simulink model "Traj2"  (R2025b)
settings: Solver=VariableStepAuto  StartTime=0.0  StopTime=T_end  RelTol=1e-3
values from neighbouring files (symbols this model uses):
  K = lqr(A, B, Q, R)    [lq.m]    (also in lqr.m = lqr(A,B,Q,R))
  L = 0.4    [lq.m]    (also in lqr.m = 0.2)
  P = double(P)    [lq.m]    (also in lqr.m)
  theta0 = double(theta0)    [lq.m]    (also in lqr.m)
  theta_ref_unwrapped = double(theta_ref_unwrapped(:))    [lq.m]
  Ts_ref = double(Ts_ref)    [lq.m]    (also in lqr.m)
  vd_ref = double(vd_ref(:))    [lq.m]    (also in lqr.m)
  wd_ref = double(wd_ref(:))    [lq.m]    (also in lqr.m)
  x0 = double(x0)    [lq.m]    (also in lqr.m)
  y0 = double(y0)    [lq.m]    (also in lqr.m)
libraries: slpidlib x2
settings Model: Creator=mwali  LastModifiedBy=mwali

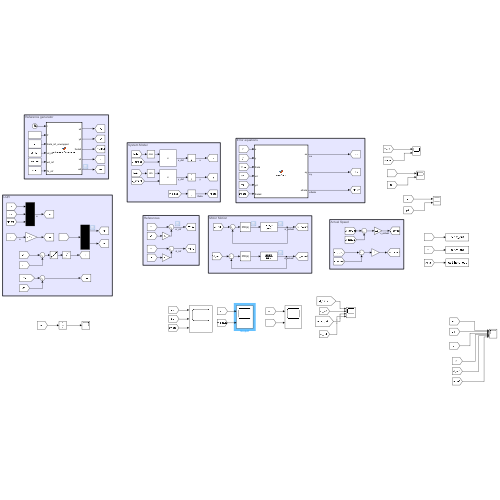
[thumbnail: Simulink's stored preview of the top-level diagram]
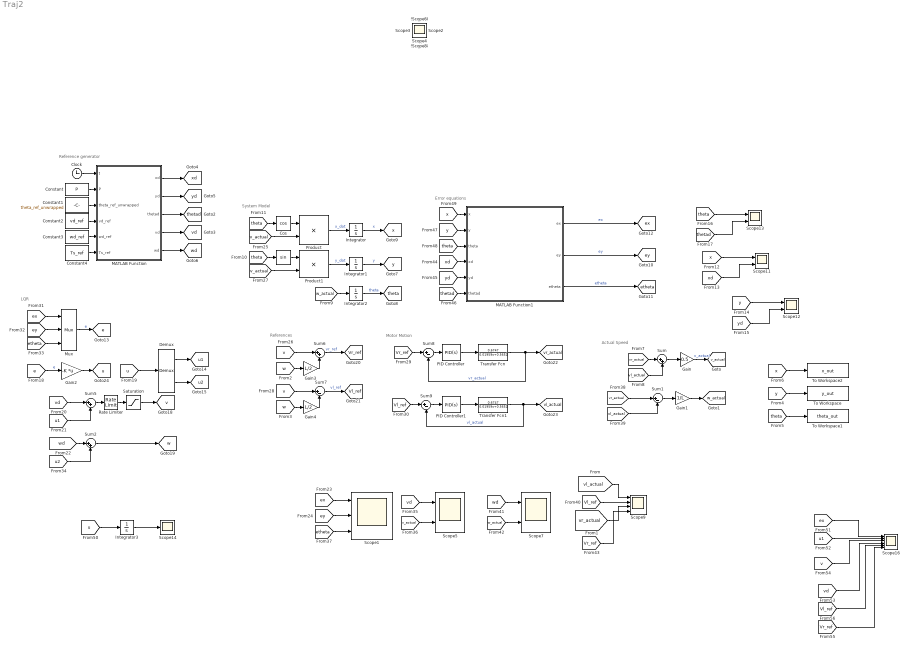
== system Traj2 ==
  note: Error equations
  note: Actual Speed
  note: Motor Motion
  note: References
  note: LQR
  note: System Model
  note: Reference generator
  " " : Trigonometry
  Clock : Clock
  Constant : Constant  Value=P
  Constant1 : Constant  Value=theta_ref_unwrapped
  Constant2 : Constant  Value=vd_ref
  Constant3 : Constant  Value=wd_ref
  Constant4 : Constant  Value=Ts_ref
  Cos : Trigonometry  Operator=cos
  Demux : Demux  Outputs=2
  Gain : Gain  Gain=0.5
  Gain1 : Gain  Gain=1/L
  Gain2 : Gain  Gain=-K  Multiplication=Matrix(K*u)
  Gain3 : Gain  Gain=L/2
  Gain4 : Gain  Gain=L/2
  Integrator : Integrator  InitialCondition=x0
  Integrator1 : Integrator  InitialCondition=y0
  Integrator2 : Integrator  InitialCondition=theta0
  Integrator3 : Integrator
  MATLAB Function : MATLAB Function  TreatAsAtomicUnit=on
  MATLAB Function1 : MATLAB Function  TreatAsAtomicUnit=on
  Mux : Mux  Inputs=3
  PID Controller : slpidlib/PID Controller  Controller=PID  Form=Parallel  TimeDomain=Continuous-time  UseExternalTs=off  SampleTime=-1  IntegratorMethod=Forward Euler  FilterMethod=Forward Euler  ControllerParametersSource=internal  P=4  I=0.05  UseKiTs=off  D=0  UseExternalDerivativeSource=off  N=100  UseFilter=on  TunerSelectOption=Transfer Function Based (PID Tuner App)  InitialConditionSource=internal  InitialConditionForIntegrator=0  InitialConditionForFilter=0  DifferentiatorICPrevScaledInput=0  ExternalReset=none  TrackingMode=off  Kt=1  LimitOutput=off  SatLimitsSource=internal  UpperSaturationLimit=0.5  LowerSaturationLimit=0  LinearizeAsGain=on  AntiWindupMode=clamping  Kb=1  LimitIntegrator=off  UpperIntegratorSaturationLimit=inf  LowerIntegratorSaturationLimit=-inf  POutMin=[]  POutMax=[]  IOutMin=[]  IOutMax=[]  DOutMin=[]  DOutMax=[]  NOutMin=[]  NOutMax=[]  SumOutMin=[]  SumOutMax=[]  SaturationOutMin=[]  SaturationOutMax=[]  PParamMin=[]  PParamMax=[]  IParamMin=[]  IParamMax=[]  DParamMin=[]  DParamMax=[]  NParamMin=[]  NParamMax=[]  KbParamMin=[]  KbParamMax=[]  KtParamMin=[]  KtParamMax=[]  KbOutMin=[]  KbOutMax=[]  KtOutMin=[]  KtOutMax=[]  IntegratorOutMin=[]  IntegratorOutMax=[]  FilterOutMin=[]  FilterOutMax=[]  SumI1OutMin=[]  SumI1OutMax=[]  SumI2OutMin=[]  SumI2OutMax=[]  SumI3OutMin=[]  SumI3OutMax=[]  SumI4OutMin=[]  SumI4OutMax=[]  SumDOutMin=[]  SumDOutMax=[]  DifferentiatorOutMin=[]  DifferentiatorOutMax=[]  FilterDiffOutCoefMin=[]  FilterDiffOutCoefMax=[]  ReciprocalOutMin=[]  ReciprocalOutMax=[]  SumDenOutMin=[]  SumDenOutMax=[]  SumNumOutMin=[]  SumNumOutMax=[]  DivideOutMin=[]  DivideOutMax=[]  UdiffTsProdOutMin=[]  UdiffTsProdOutMax=[]  NTsProdOutMin=[]  NTsProdOutMax=[]  UintegralTsProdOutMin=[]  UintegralTsProdOutMax=[]  UngainTsProdOutMin=[]  UngainTsProdOutMax=[]  ClampingZeroOutDataTypeStr=Inherit: Inherit via back propagation  ClampingZeroOutMin=[]  ClampingZeroOutMax=[]  FilterDenConstantOutDataTypeStr=Inherit: Inherit via back propagation  FilterDenConstantOutMin=[]  FilterDenConstantOutMax=[]  PCopyOutDataTypeStr=Inherit: Inherit via back propagation  PCopyOutMin=[]  PCopyOutMax=[]  NCopyOutDataTypeStr=Inherit: Inherit via back propagation  NCopyOutMin=[]  NCopyOutMax=[]  IntegratorContinuousStateAttributes=''  IntegratorStateMustResolveToSignalObject=off  IntegratorRTWStateStorageClass=Auto  FilterContinuousStateAttributes=''  FilterStateMustResolveToSignalObject=off  FilterRTWStateStorageClass=Auto  ParallelPVariant=InternalParameters  IdealPVariant=Disabled  IVariant=InternalParameters  DVariant=InternalParameters  IntegratorVariant=Continuous  SatVariant=Disabled  AWVariant=Passthrough  PCopyVariant=Disabled  TRVariant=Disabled  FdbkBlocksVariant=Forward  IdealPFdbkVariant=Disabled  SatFdbkVariant=Disabled  DerivativeFilterVariant=ContFilter  NVariant=InternalParameters  NCopyVariant=Disabled  FilterICVariant=InternalICsFilter  IntegratorICVariant=InternalICs  ExternalResetVariant=Disabled  TRSumVariant=Passthrough  SumFdbkVariant=Disabled  SumVariant=Sum_PID  TsampFilterVariant=InternalTs  TsampNgainVariant=Passthrough  TsampIntegralVariant=Disabled_SignalSpec  ExternalSaturationOutDataTypeStr=Inherit: Same as second input  DerivativeSourceVariant=ErrorSignal  PreIntVariant=InternalPreInt
  PID Controller1 : slpidlib/PID Controller  Controller=PID  Form=Parallel  TimeDomain=Continuous-time  UseExternalTs=off  SampleTime=-1  IntegratorMethod=Forward Euler  FilterMethod=Forward Euler  ControllerParametersSource=internal  P=4  I=0.05  UseKiTs=off  D=0  UseExternalDerivativeSource=off  N=100  UseFilter=on  TunerSelectOption=Transfer Function Based (PID Tuner App)  InitialConditionSource=internal  InitialConditionForIntegrator=0  InitialConditionForFilter=0  DifferentiatorICPrevScaledInput=0  ExternalReset=none  TrackingMode=off  Kt=1  LimitOutput=off  SatLimitsSource=internal  UpperSaturationLimit=0.5  LowerSaturationLimit=0  LinearizeAsGain=on  AntiWindupMode=clamping  Kb=1  LimitIntegrator=off  UpperIntegratorSaturationLimit=inf  LowerIntegratorSaturationLimit=-inf  POutMin=[]  POutMax=[]  IOutMin=[]  IOutMax=[]  DOutMin=[]  DOutMax=[]  NOutMin=[]  NOutMax=[]  SumOutMin=[]  SumOutMax=[]  SaturationOutMin=[]  SaturationOutMax=[]  PParamMin=[]  PParamMax=[]  IParamMin=[]  IParamMax=[]  DParamMin=[]  DParamMax=[]  NParamMin=[]  NParamMax=[]  KbParamMin=[]  KbParamMax=[]  KtParamMin=[]  KtParamMax=[]  KbOutMin=[]  KbOutMax=[]  KtOutMin=[]  KtOutMax=[]  IntegratorOutMin=[]  IntegratorOutMax=[]  FilterOutMin=[]  FilterOutMax=[]  SumI1OutMin=[]  SumI1OutMax=[]  SumI2OutMin=[]  SumI2OutMax=[]  SumI3OutMin=[]  SumI3OutMax=[]  SumI4OutMin=[]  SumI4OutMax=[]  SumDOutMin=[]  SumDOutMax=[]  DifferentiatorOutMin=[]  DifferentiatorOutMax=[]  FilterDiffOutCoefMin=[]  FilterDiffOutCoefMax=[]  ReciprocalOutMin=[]  ReciprocalOutMax=[]  SumDenOutMin=[]  SumDenOutMax=[]  SumNumOutMin=[]  SumNumOutMax=[]  DivideOutMin=[]  DivideOutMax=[]  UdiffTsProdOutMin=[]  UdiffTsProdOutMax=[]  NTsProdOutMin=[]  NTsProdOutMax=[]  UintegralTsProdOutMin=[]  UintegralTsProdOutMax=[]  UngainTsProdOutMin=[]  UngainTsProdOutMax=[]  ClampingZeroOutDataTypeStr=Inherit: Inherit via back propagation  ClampingZeroOutMin=[]  ClampingZeroOutMax=[]  FilterDenConstantOutDataTypeStr=Inherit: Inherit via back propagation  FilterDenConstantOutMin=[]  FilterDenConstantOutMax=[]  PCopyOutDataTypeStr=Inherit: Inherit via back propagation  PCopyOutMin=[]  PCopyOutMax=[]  NCopyOutDataTypeStr=Inherit: Inherit via back propagation  NCopyOutMin=[]  NCopyOutMax=[]  IntegratorContinuousStateAttributes=''  IntegratorStateMustResolveToSignalObject=off  IntegratorRTWStateStorageClass=Auto  FilterContinuousStateAttributes=''  FilterStateMustResolveToSignalObject=off  FilterRTWStateStorageClass=Auto  ParallelPVariant=InternalParameters  IdealPVariant=Disabled  IVariant=InternalParameters  DVariant=InternalParameters  IntegratorVariant=Continuous  SatVariant=Disabled  AWVariant=Passthrough  PCopyVariant=Disabled  TRVariant=Disabled  FdbkBlocksVariant=Forward  IdealPFdbkVariant=Disabled  SatFdbkVariant=Disabled  DerivativeFilterVariant=ContFilter  NVariant=InternalParameters  NCopyVariant=Disabled  FilterICVariant=InternalICsFilter  IntegratorICVariant=InternalICs  ExternalResetVariant=Disabled  TRSumVariant=Passthrough  SumFdbkVariant=Disabled  SumVariant=Sum_PID  TsampFilterVariant=InternalTs  TsampNgainVariant=Passthrough  TsampIntegralVariant=Disabled_SignalSpec  ExternalSaturationOutDataTypeStr=Inherit: Same as second input  DerivativeSourceVariant=ErrorSignal  PreIntVariant=InternalPreInt
  Product : Product
  Product1 : Product
  Rate Limiter : RateLimiter  RisingSlewLimit=0.1  FallingSlewLimit=-0.35  SampleTimeMode=inherited
  Saturation : Saturate  UpperLimit=0.3  LowerLimit=0
  Scope1 : Scope  NumInputPorts=3
      settings: ActiveDisplayYMinimum=-0.19694  ActiveDisplayYMaximum=0.26619
  Scope{5,7,11..13} (5 alike) : Scope  NumInputPorts=2
      Scope11 settings: ActiveDisplayYMinimum=-1  ActiveDisplayYMaximum=1  DataLoggingVariableName=ScopeData11
      Scope12 settings: ActiveDisplayYMinimum=-1  ActiveDisplayYMaximum=1  DataLoggingVariableName=ScopeData12
      Scope13 settings: ActiveDisplayYMinimum=1.0311287515557852  ActiveDisplayYMaximum=3.7167864278411562  DataLoggingVariableName=ScopeData13
      Scope5 settings: ActiveDisplayYMinimum=-0.041698068879938432  ActiveDisplayYMaximum=0.34024051073415013  DataLoggingVariableName=ScopeData5
      Scope7 settings: ActiveDisplayYMinimum=-2.7766  ActiveDisplayYMaximum=4.0045  DataLoggingVariableName=ScopeData7
  Scope{,2..4,6,8,10,14..15} (9 alike) : Scope
      Scope14 settings: ActiveDisplayYMinimum=-1  ActiveDisplayYMaximum=1  DataLoggingVariableName=ScopeData14
      Scope settings: ActiveDisplayYMinimum=-0.11929  ActiveDisplayYMaximum=0.80552
      Scope10 settings: ActiveDisplayYMinimum=-1  ActiveDisplayYMaximum=1  DataLoggingVariableName=ScopeData10
      Scope15 settings: ActiveDisplayYMinimum=-1  ActiveDisplayYMaximum=1  DataLoggingVariableName=ScopeData15
      Scope2 settings: ActiveDisplayYMinimum=-1  ActiveDisplayYMaximum=1  DataLoggingVariableName=ScopeData2
      Scope3 settings: ActiveDisplayYMinimum=-1  ActiveDisplayYMaximum=1  DataLoggingVariableName=ScopeData3
      Scope4 settings: ActiveDisplayYMinimum=-1  ActiveDisplayYMaximum=1  DataLoggingVariableName=ScopeData4
      Scope6 settings: ActiveDisplayYMinimum=-1  ActiveDisplayYMaximum=1  DataLoggingVariableName=ScopeData6
      Scope8 settings: ActiveDisplayYMinimum=-5.1687  ActiveDisplayYMaximum=3.6193  DataLoggingVariableName=ScopeData8
  Scope16 : Scope  NumInputPorts=6
      settings: ActiveDisplayYMinimum=-0.13161054609059852  ActiveDisplayYMaximum=0.33829750120743474  DataLoggingVariableName=ScopeData16
  Scope9 : Scope  NumInputPorts=4
      settings: ActiveDisplayYMinimum=-0.51559  ActiveDisplayYMaximum=1.245  DataLoggingVariableName=ScopeData9
  Sum{,2,5..6} (4 alike) : Sum  Inputs=|++
  Sum{1,7..9} (4 alike) : Sum  Inputs=|+-
  To Workspace : ToWorkspace  VariableName=y_out  SampleTime=-1
  To Workspace1 : ToWorkspace  VariableName=theta_out  SampleTime=-1
  To Workspace2 : ToWorkspace  VariableName=x_out  SampleTime=-1
  Transfer Fcn : TransferFcn  Numerator=[0.6747]  Denominator=[0.01959 0.5652]
  Transfer Fcn1 : TransferFcn  Numerator=[0.6747]  Denominator=[0.01959 0.5652]
  tag scope: Vl_ref=global, Vr_ref=global, e=global, etheta=global, ex=global, ey=global, theta=global, thetad=global, u1=global, u2=global, u=global, v=global, v_actual=global, vd=global, vl_actual=global, vr_actual=global, w=global, w_actual=global, wd=global, x=global, xd=global, y=global, yd=global
  wires:
  [y] -> To Workspace/1
  [theta] -> To Workspace1/1
  [x] -> To Workspace2/1
  [vd] -> Scope5/1
  [v_actual] -> Scope5/2
  [wd] -> Scope7/1
  [w_actual] -> Scope7/2
  [ex] -> Scope1/1
  [ey] -> Scope1/2
  [etheta] -> Scope1/3
  [vl_actual] -> Scope9/1
  [vr_actual] -> Scope9/3
  Constant/1 -> MATLAB Function/2(P)
  Constant2/1 -> MATLAB Function/4(vd_ref)
  Clock/1 -> MATLAB Function/1(t)
  MATLAB Function/4(vd) -> [vd]
  Constant1/1 -> MATLAB Function/3(theta_ref_unwrapped)
  MATLAB Function/5(wd) -> [wd]
  MATLAB Function/3(thetad) -> [thetad]
  Constant4/1 -> MATLAB Function/6(Ts_ref)
  MATLAB Function/2(yd) -> [yd]
  MATLAB Function/1(xd) -> [xd]
  Constant3/1 -> MATLAB Function/5(wd_ref)
  [theta] -> " "/1
  " "/1 -> Product1/1
  Integrator/1 -> [x]  "x"
  Cos/1 -> Product/1
  Integrator2/1 -> [theta]  "theta"
  Product1/1 -> Integrator1/1  "y_dot"
  [w_actual] -> Integrator2/1
  Product/1 -> Integrator/1  "x_dot"
  [v_actual] -> Product/2
  [v_actual] -> Product1/2
  Integrator1/1 -> [y]  "y"
  [theta] -> Cos/1
  [e] -> Gain2/1  "e"
  [u1] -> Sum5/2
  Sum5/1 -> Rate Limiter/1
  [ey] -> Mux/2
  [ex] -> Mux/1
  [wd] -> Sum2/1
  Mux/1 -> [e]  "e"
  [etheta] -> Mux/3
  Demux/1 -> [u1]
  [u2] -> Sum2/2
  Gain2/1 -> [u]
  [vd] -> Sum5/1
  Demux/2 -> [u2]
  Sum2/1 -> [w]
  [u] -> Demux/1
  [v] -> Sum7/1
  [w] -> Gain4/1
  Sum6/1 -> [Vr_ref]  "vr_ref"
  Gain4/1 -> Sum7/2
  [w] -> Gain3/1
  [v] -> Sum6/1
  Sum7/1 -> [Vl_ref]  "vl_ref"
  Gain3/1 -> Sum6/2
  Sum8/1 -> PID Controller/1
  Transfer Fcn/1 -> [vr_actual], Sum8/2  "vr_actual"
  [Vr_ref] -> Sum8/1
  [Vl_ref] -> Sum9/1
  PID Controller1/1 -> Transfer Fcn1/1
  Sum9/1 -> PID Controller1/1
  Transfer Fcn1/1 -> [vl_actual], Sum9/2  "vl_actual"
  PID Controller/1 -> Transfer Fcn/1
  Gain1/1 -> [w_actual]
  [vr_actual] -> Sum/1
  Gain/1 -> [v_actual]  "v_actual"
  Sum/1 -> Gain/1
  [vr_actual] -> Sum1/1
  [vl_actual] -> Sum/2
  [vl_actual] -> Sum1/2
  Sum1/1 -> Gain1/1
  [Vl_ref] -> Scope9/2
  [Vr_ref] -> Scope9/4
  [x] -> Scope11/1
  [xd] -> Scope11/2
  [y] -> Scope12/1
  [yd] -> Scope12/2
  [theta] -> Scope13/1
  [thetad] -> Scope13/2
  [thetad] -> MATLAB Function1/6(thetad)
  MATLAB Function1/2(ey) -> [ey]  "ey"
  MATLAB Function1/3(etheta) -> [etheta]  "etheta"
  [x] -> MATLAB Function1/1(x)
  [yd] -> MATLAB Function1/5(yd)
  [xd] -> MATLAB Function1/4(xd)
  [y] -> MATLAB Function1/2(y)
  MATLAB Function1/1(ex) -> [ex]  "ex"
  [theta] -> MATLAB Function1/3(theta)
  [u] -> Integrator3/1
  Integrator3/1 -> Scope14/1
  [ex] -> Scope16/1
  [u1] -> Scope16/2
  [v] -> Scope16/3
  [vd] -> Scope16/4
  [Vl_ref] -> Scope16/5
  [Vr_ref] -> Scope16/6
  Rate Limiter/1 -> Saturation/1
  Saturation/1 -> [v]

== matlab function Traj2/MATLAB Function1 ==
  data: x input; ex output; y input; theta input; xd input; yd input; thetad input; ey output; etheta output
function [ex, ey, etheta] = calcError(x, y, theta, xd, yd, thetad)

dx = x - xd;
dy = y - yd;

ex =  cos(thetad)*dx + sin(thetad)*dy;
ey = -sin(thetad)*dx + cos(thetad)*dy;

etheta = atan2(sin(theta - thetad), cos(theta - thetad));

== matlab function Traj2/MATLAB Function ==
  data: t input; P input; theta_ref_unwrapped input; vd_ref input; wd_ref input; Ts_ref input; xd output; yd output; thetad output; vd output; wd output
function [xd, yd, thetad, vd, wd] = referenceGenerator(t, P, theta_ref_unwrapped, vd_ref, wd_ref, Ts_ref)

t_vec = (0:size(P,1)-1)' * Ts_ref;

% ===== Safe startup timing =====
T_hold = 1;   % keep reference fixed at the start
T_soft = 3;   % then release it gradually
beta0  = 0.25;  % initial reference speed = 25% of normal

if t <= T_hold
    t_eff = 0;

elseif t <= (T_hold + T_soft)
    dt  = t - T_hold;
    tau = dt / T_soft;   % 0 -> 1

    % Integrated smooth speed scaling
    % This guarantees dt_eff/dt stays between beta0 and 1
    t_eff = beta0*dt + (1 - beta0)*T_soft*(tau^3 - 0.5*tau^4);

else
    t_soft_end = T_soft * (0.5 + 0.5*beta0);
    t_eff = t_soft_end + (t - T_hold - T_soft);
end

% Clamp time
t_clamped = min(max(t_eff, 0), t_vec(end));

% Interpolate reference
xd     = interp1(t_vec, P(:,1), t_clamped, 'linear');
yd     = interp1(t_vec, P(:,2), t_clamped, 'linear');
thetad = interp1(t_vec, theta_ref_unwrapped, t_clamped, 'linear');
vd     = interp1(t_vec, vd_ref, t_clamped, 'linear');
wd     = interp1(t_vec, wd_ref, t_clamped, 'linear');

vd = max(vd, 0);
